simulink model "sensor"  (R2018a)
settings: Solver=FixedStepAuto  StartTime=0.0  StopTime=time_end  FixedStep=dt  RelTol=1e-3
values from neighbouring files (symbols this model uses):
  tau = 1/(2*pi*0.2)    (= 0.795774715459)    [sim_sensor.m]    (also in sim_sensor_2.m)
settings Model: Creator=aoki-soya  LastModifiedBy=aoki-soya

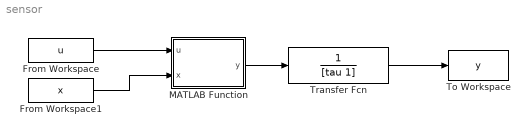
== system sensor ==
  From Workspace : FromWorkspace  VariableName=u  SampleTime=0
  From Workspace1 : FromWorkspace  VariableName=x  SampleTime=0
  MATLAB Function : MATLAB Function  TreatAsAtomicUnit=on
  To Workspace : ToWorkspace  VariableName=y  SaveFormat=Timeseries  SampleTime=-1
  Transfer Fcn : TransferFcn  Denominator=[tau 1]
  wires:
  From Workspace/1 -> MATLAB Function/1(u)
  From Workspace1/1 -> MATLAB Function/2(x)
  MATLAB Function/1(y) -> Transfer Fcn/1
  Transfer Fcn/1 -> To Workspace/1

== matlab function sensor/MATLAB Function ==
  settings: updateMethod=DISCRETE  sampleTime=dt
  data: u input; y output; x input
function y = sensor(u,x)

% mu & sigma
% 固定値版、GPにするならここを変える
mu = 0;
sigma = 0;
if (abs(u) < 15)
    mu = 0.2482;
    sigma = 0.3364;
elseif ((15 <= abs(u)) && (abs(u) < 30))
    mu = 1.3709;
    sigma = 1.3709;
elseif (30 <= abs(u))
    mu = 3.2910;
    sigma = 0.4885;
end

y = normrnd(sign(u)*(abs(u)+mu), sigma);
